simulink model "final_test1"  (Simulink 7.7)
settings: Solver=ode45  StartTime=0.0  StopTime=10.0  RelTol=1e-3
undefined symbols (not defined in the file): des_attributefunction_support, des_figposition
libraries: simeventsattributes2 x107, simeventsserver1 x73, simeventstranslate1 x43, simeventsrouting1 x28, commrandsrc2 x18, simeventsgenerators1 x12, simeventssink1 x9, simeventsqueue1 x6, simulink_extras x1, simeventssignalmanage1 x1
(part 5 of 5)

== matlab function Green Link/Attribute Function/Embedded MATLAB Function ==
  data: length input double; out_ServiceTime output double
  events: trigger input FUNCTION_CALL_EVENT
function out_ServiceTime= fcn(length)
%FCN    Access and modify attributes with MATLAB 
% 
% Input arguments must match the attribute names.
% Output arguments must be out_<AttributeName>,
% e.g., out_ServiceTime where ServiceTime is the attribute name.
% 
% The output attribute will be created if it is not present.
%

cap = 3.0 * 1024 * 1024;
out_ServiceTime = length/cap;

== matlab function Green Link/Attribute Function1/Embedded MATLAB Function ==
  data: length input double; out_ServiceTime output double
  events: trigger input FUNCTION_CALL_EVENT
function out_ServiceTime  = fcn(length)
%FCN    Access and modify attributes with MATLAB 
% 
% Input arguments must match the attribute names.
% Output arguments must be out_<AttributeName>,
% e.g., out_ServiceTime where ServiceTime is the attribute name.
% 
% The output attribute will be created if it is not present.
%

cap = 3.0 * 1024 * 1024;
out_ServiceTime = length/cap;

== matlab function Green Link1/Attribute Function/Embedded MATLAB Function ==
  data: length input double; out_ServiceTime output double
  events: trigger input FUNCTION_CALL_EVENT
function out_ServiceTime= fcn(length)
%FCN    Access and modify attributes with MATLAB 
% 
% Input arguments must match the attribute names.
% Output arguments must be out_<AttributeName>,
% e.g., out_ServiceTime where ServiceTime is the attribute name.
% 
% The output attribute will be created if it is not present.
%

cap = 3.0 * 1024 * 1024;
out_ServiceTime = length/cap;

== matlab function Green Link1/Attribute Function1/Embedded MATLAB Function ==
  data: length input double; out_ServiceTime output double
  events: trigger input FUNCTION_CALL_EVENT
function out_ServiceTime  = fcn(length)
%FCN    Access and modify attributes with MATLAB 
% 
% Input arguments must match the attribute names.
% Output arguments must be out_<AttributeName>,
% e.g., out_ServiceTime where ServiceTime is the attribute name.
% 
% The output attribute will be created if it is not present.
%

cap = 3.0 * 1024 * 1024;
out_ServiceTime = length/cap;

== matlab function Green Link2/Attribute Function/Embedded MATLAB Function ==
  data: length input double; out_ServiceTime output double
  events: trigger input FUNCTION_CALL_EVENT
function out_ServiceTime= fcn(length)
%FCN    Access and modify attributes with MATLAB 
% 
% Input arguments must match the attribute names.
% Output arguments must be out_<AttributeName>,
% e.g., out_ServiceTime where ServiceTime is the attribute name.
% 
% The output attribute will be created if it is not present.
%

cap = 3.0 * 1024 * 1024;
out_ServiceTime = length/cap;

== matlab function Green Link2/Attribute Function1/Embedded MATLAB Function ==
  data: length input double; out_ServiceTime output double
  events: trigger input FUNCTION_CALL_EVENT
function out_ServiceTime  = fcn(length)
%FCN    Access and modify attributes with MATLAB 
% 
% Input arguments must match the attribute names.
% Output arguments must be out_<AttributeName>,
% e.g., out_ServiceTime where ServiceTime is the attribute name.
% 
% The output attribute will be created if it is not present.
%

cap = 3.0 * 1024 * 1024;
out_ServiceTime = length/cap;

== matlab function Green Link3/Attribute Function/Embedded MATLAB Function ==
  data: length input double; out_ServiceTime output double
  events: trigger input FUNCTION_CALL_EVENT
function out_ServiceTime= fcn(length)
%FCN    Access and modify attributes with MATLAB 
% 
% Input arguments must match the attribute names.
% Output arguments must be out_<AttributeName>,
% e.g., out_ServiceTime where ServiceTime is the attribute name.
% 
% The output attribute will be created if it is not present.
%

cap = 3.0 * 1024 * 1024;
out_ServiceTime = length/cap;

== matlab function Green Link3/Attribute Function1/Embedded MATLAB Function ==
  data: length input double; out_ServiceTime output double
  events: trigger input FUNCTION_CALL_EVENT
function out_ServiceTime  = fcn(length)
%FCN    Access and modify attributes with MATLAB 
% 
% Input arguments must match the attribute names.
% Output arguments must be out_<AttributeName>,
% e.g., out_ServiceTime where ServiceTime is the attribute name.
% 
% The output attribute will be created if it is not present.
%

cap = 3.0 * 1024 * 1024;
out_ServiceTime = length/cap;

== matlab function Green Link4/Attribute Function/Embedded MATLAB Function ==
  data: length input double; out_ServiceTime output double
  events: trigger input FUNCTION_CALL_EVENT
function out_ServiceTime= fcn(length)
%FCN    Access and modify attributes with MATLAB 
% 
% Input arguments must match the attribute names.
% Output arguments must be out_<AttributeName>,
% e.g., out_ServiceTime where ServiceTime is the attribute name.
% 
% The output attribute will be created if it is not present.
%

cap = 3.0 * 1024 * 1024;
out_ServiceTime = length/cap;

== matlab function Green Link4/Attribute Function1/Embedded MATLAB Function ==
  data: length input double; out_ServiceTime output double
  events: trigger input FUNCTION_CALL_EVENT
function out_ServiceTime  = fcn(length)
%FCN    Access and modify attributes with MATLAB 
% 
% Input arguments must match the attribute names.
% Output arguments must be out_<AttributeName>,
% e.g., out_ServiceTime where ServiceTime is the attribute name.
% 
% The output attribute will be created if it is not present.
%

cap = 3.0 * 1024 * 1024;
out_ServiceTime = length/cap;

== matlab function Host 1/Attribute Function/Embedded MATLAB Function ==
  data: type input double; out_length output double; size input double
  events: trigger input FUNCTION_CALL_EVENT
function out_length  = fcn(type, size)
base = 256;
if (type == 1)
    base = 512;
end
out_length = base * 2^size * 8;

== matlab function Host 2/Attribute Function/Embedded MATLAB Function ==
  data: type input double; out_length output double; size input double
  events: trigger input FUNCTION_CALL_EVENT
function out_length  = fcn(type, size)
base = 256;
if (type == 1)
    base = 512;
end
out_length = base * 2^size * 8;

== matlab function Host 3/Attribute Function/Embedded MATLAB Function ==
  data: type input double; out_length output double; size input double
  events: trigger input FUNCTION_CALL_EVENT
function out_length  = fcn(type, size)
base = 256;
if (type == 1)
    base = 512;
end
out_length = base * 2^size * 8;

== matlab function Host 4/Attribute Function/Embedded MATLAB Function ==
  data: type input double; out_length output double; size input double
  events: trigger input FUNCTION_CALL_EVENT
function out_length  = fcn(type, size)
base = 256;
if (type == 1)
    base = 512;
end
out_length = base * 2^size * 8;

== matlab function Host 5/Attribute Function/Embedded MATLAB Function ==
  data: type input double; out_length output double; size input double
  events: trigger input FUNCTION_CALL_EVENT
function out_length  = fcn(type, size)
base = 256;
if (type == 1)
    base = 512;
end
out_length = base * 2^size * 8;

== matlab function Host 6/Attribute Function/Embedded MATLAB Function ==
  data: type input double; out_length output double; size input double
  events: trigger input FUNCTION_CALL_EVENT
function out_length  = fcn(type, size)
base = 256;
if (type == 1)
    base = 512;
end
out_length = base * 2^size * 8;
